simulink model "intregral"  (R2017b)
settings: Solver=VariableStepAuto  StartTime=0.0  StopTime=10.0  RelTol=1e-3
settings Model: Creator=MY  LastModifiedBy=MY

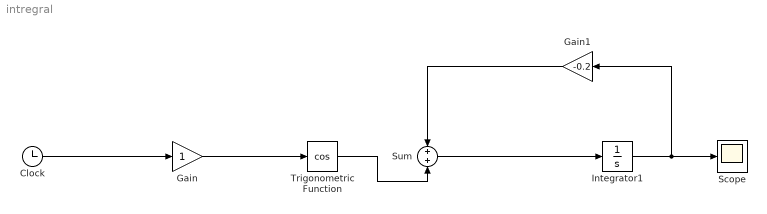
== system intregral ==
  Clock : Clock
  Gain : Gain
  Gain1 : Gain  Gain=-0.2
  Integrator1 : Integrator
  Scope : Scope
  Sum : Sum
  Trigonometric Function : Trigonometry  Operator=cos
  wires:
  Clock/1 -> Gain/1
  Gain/1 -> Trigonometric Function/1
  Sum/1 -> Integrator1/1
  Integrator1/1 -> Gain1/1, Scope/1
  Gain1/1 -> Sum/1
  Trigonometric Function/1 -> Sum/2
